simulink model "telemetry"  (Simulink 7.2)
settings: Solver=ode45  StartTime=0.0  StopTime=10.0  RelTol=1e-3
libraries: dsparch4 x7, commchan3 x1, commrandsrc2 x1, commsynccomp2 x1, dspmlti4 x1, commfilt2 x1
settings Model: Creator=student  LastModifiedBy=student
settings DebuggingCC: AlgebraicLoopMsg=none  SolverPrmCheckMsg=none  UnconnectedInputMsg=none  UnconnectedOutputMsg=none  UnconnectedLineMsg=none

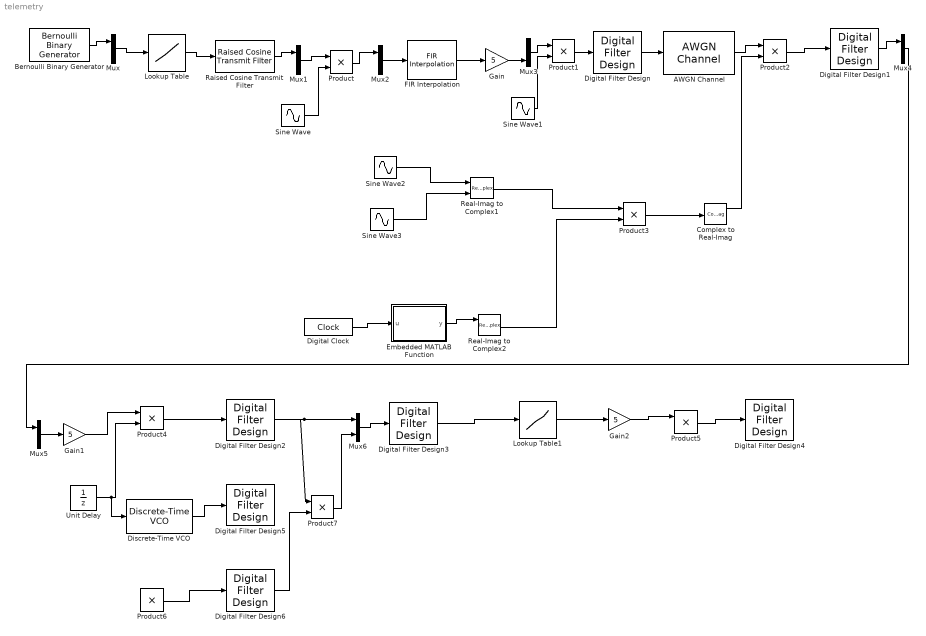
== system telemetry ==
  AWGN Channel : commchan3/AWGN Channel  SystemSampleTime=-1  seed=67  noiseMode="Signal to noise ratio  (Eb/No)"  EbNodB=10  EsNodB=10  SNRdB=10  bitsPerSym=1  Ps=1  Tsym=1  variance=1
  Bernoulli Binary Generator : commrandsrc2/Bernoulli Binary Generator  DialogController=commDDGCreate  DialogControllerArgs=DataTag0  SystemSampleTime=-1  P=0.5  seed=61  Ts=1  frameBased=off  sampPerFrame=1  orient=off  outDataType=double
  Complex to Real-Imag : ComplexToRealImag
  Digital Filter Design{,1..6} (7 alike) : dsparch4/Digital Filter Design  SystemSampleTime=-1  mwdsp_browser_bugfix_var=off
  Digital Clock : DigitalClock
  Discrete-Time VCO : commsynccomp2/Discrete-Time VCO  SystemSampleTime=-1  Ac=1  Fc=10  Kc=1  Ph=0  ts=0.01
  Embedded MATLAB Function : Stateflow chart
  FIR Interpolation : dspmlti4/FIR Interpolation  DialogController=dspdialog.FIRInterpolation  DialogControllerArgs=DataTag8  h=fir1(15,1/4)  L=3  framing=Maintain input frame size  outputBufInitCond=0  roundingMode=Floor  overflowMode=off  FilterSource=Specify via dialog  FilterObject=Hm_firinterp
  Gain : Gain  Gain=5  ParameterDataType=sfix(16)  ParameterScaling=2^0  OutDataType=sfix(16)  OutScaling=2^0
  Gain1 : Gain  Gain=5  ParameterDataType=sfix(16)  ParameterScaling=2^0  OutDataType=sfix(16)  OutScaling=2^0
  Gain2 : Gain  Gain=5  ParameterDataType=sfix(16)  ParameterScaling=2^0  OutDataType=sfix(16)  OutScaling=2^0
  Lookup Table : Lookup  InputValues=[-5:5]  Table=tanh([-5:5])  OutDataType=sfix(16)  OutScaling=2^0
  Lookup Table1 : Lookup  InputValues=[-5:5]  Table=tanh([-5:5])  OutDataType=sfix(16)  OutScaling=2^0
  Mux{,1..6} (7 alike) : Mux  Inputs=2
  Product{,1..7} (8 alike) : Product  OutDataType=sfix(16)  OutScaling=2^0  RndMeth=Zero
  Raised Cosine Transmit Filter : commfilt2/Raised Cosine Transmit Filter  DialogController=dspDDGCreate  DialogControllerArgs=DataTag9  SystemSampleTime=-1  filtType=Square root  D=4  R=0.2  sampMode=Mute  saveAsFlag=0  framing=Maintain input frame rate  N=8  checkGain=Normalized  filterGain=1  checkCoeff=off  variableName=rcTxFilt  launchFVT=off  roundingMode=Floor  overflowMode=off
  Real-Imag to Complex1 : RealImagToComplex
  Real-Imag to Complex2 : RealImagToComplex
  Sine Wave{,1..3} (4 alike) : Sin  SampleTime=0
  Unit Delay : UnitDelay
  wires:
  Bernoulli Binary Generator/1 -> Mux/1
  Mux/1 -> Lookup Table/1
  Lookup Table/1 -> Raised Cosine Transmit Filter/1
  Raised Cosine Transmit Filter/1 -> Mux1/1
  Mux1/1 -> Product/1
  Sine Wave/1 -> Product/2
  Product/1 -> Mux2/1
  Mux2/1 -> FIR Interpolation/1
  FIR Interpolation/1 -> Gain/1
  Gain/1 -> Mux3/2
  Mux3/1 -> Product1/1
  Sine Wave1/1 -> Product1/2
  Product1/1 -> Digital Filter Design/1
  Digital Filter Design/1 -> AWGN Channel/1
  AWGN Channel/1 -> Product2/1
  Product2/1 -> Digital Filter Design1/1
  Complex to Real-Imag/1 -> Product2/2
  Product3/1 -> Complex to Real-Imag/1
  Real-Imag to Complex1/1 -> Product3/1
  Real-Imag to Complex2/1 -> Product3/2
  Sine Wave2/1 -> Real-Imag to Complex1/1
  Sine Wave3/1 -> Real-Imag to Complex1/2
  Embedded MATLAB Function/1(y) -> Real-Imag to Complex2/1
  Digital Clock/1 -> Embedded MATLAB Function/1(u)
  Digital Filter Design1/1 -> Mux4/1
  Mux4/1 -> Mux5/1
  Mux5/1 -> Gain1/1
  Gain1/1 -> Product4/1
  Product4/1 -> Digital Filter Design2/1
  Digital Filter Design2/1 -> Mux6/1, Product7/1
  Mux6/1 -> Digital Filter Design3/1
  Lookup Table1/1 -> Gain2/1
  Digital Filter Design3/1 -> Lookup Table1/1
  Gain2/1 -> Product5/1
  Product5/1 -> Digital Filter Design4/1
  Unit Delay/1 -> Product4/2, Discrete-Time VCO/1
  Product6/1 -> Digital Filter Design6/1
  Discrete-Time VCO/1 -> Digital Filter Design5/1
  Digital Filter Design6/1 -> Product7/2
  Product7/1 -> Mux6/2

== matlab function Embedded MATLAB Function ==
  data: u input double; y output double
function y = fcn(u)
% This block supports the Embedded MATLAB subset.
% See the help menu for details. 

y = u;
